simulink subsystem "Forces_and_Moments"  (R2025b)
settings: Solver=VariableStepAuto  StartTime=0.0  StopTime=10.0  RelTol=1e-3
undefined symbols (not defined in the file): canard_pos_r_mean, chute_drogue_drag, chute_drogue_time, chute_enable, chute_main_drag, chute_main_threshold, chute_main_time, rocket_diameter
settings Model: Creator=joedo  LastModifiedBy=jaiden

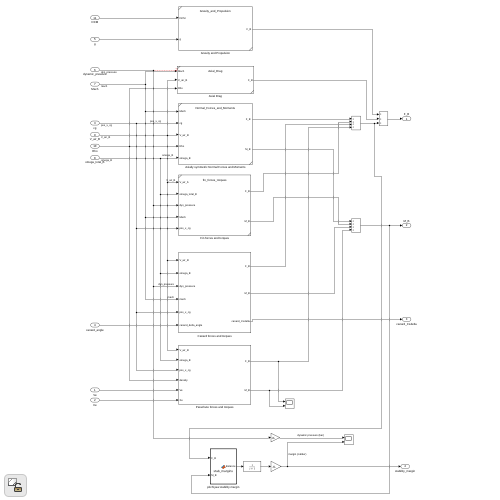
[thumbnail: Simulink's stored preview of the top-level diagram]
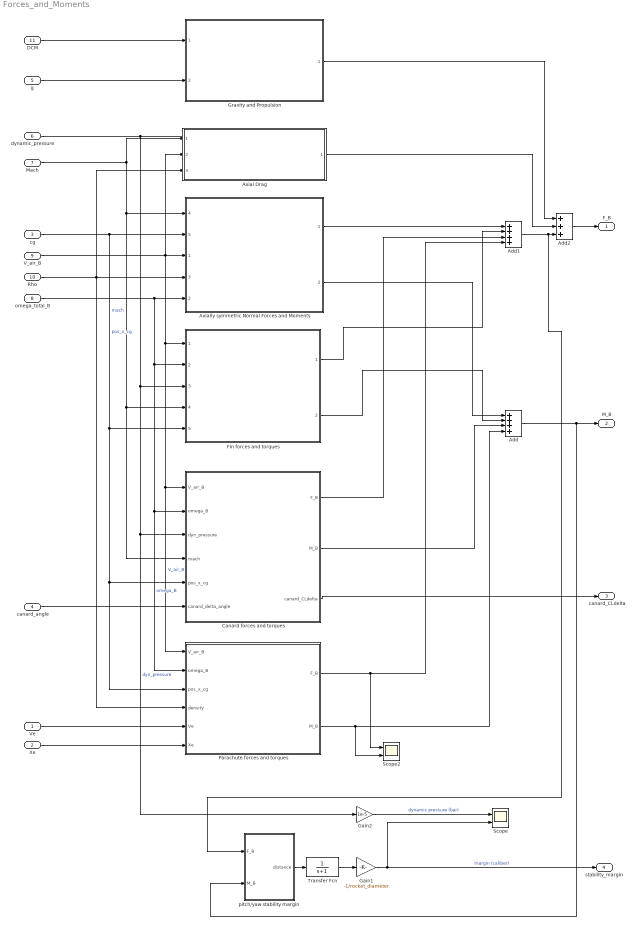
== system Forces_and_Moments ==
  Ve : Inport
  Xe : Inport  Port=2
  cg : Inport  Port=3
  canard_angle : Inport  Port=4
  g : Inport  Port=5
  "dynamic_pressure " : Inport  Port=6
  Mach : Inport  Port=7
  omega_total_B : Inport  Port=8
  V_air_B : Inport  Port=9
  Rho : Inport  Port=10
  DCM : Inport  Port=11
  Add : Sum  Inputs=++++
  Add1 : Sum  Inputs=++++
  Add2 : Sum  Inputs=+++
  Axial Drag : Subsystem  ReferencedSubsystem=Axial_Drag
  Axially symmetric Normal Forces and Moments : Subsystem  ReferencedSubsystem=Normal_Forces_and_Moments
      settings: PortSchema="{\"entries\":[{\"content\":{\"sides\":[{\"content\":{\"connectorIds\":[\"In4\",\"In5\",\"In1\",\"In3\",\"In2\"]},\"type\":\"ConnectorPlacement.EquallySpacedRectSide\",\"uuid\":\"3d060e6d-6cf3-4341-877b-3cb591774c08\"},{\"content\":{\"connectorIds\":[\"Out1\",\"Out2\"],\"side\":\"RIGHT\"},\"type\":\"ConnectorPlacement.EquallySpacedRectSide\",\"uuid\":\"12a83e93-0b1c-4946-a0d1-6eef9ce0d7d5\"},{\"content\":{\"side\":\"TOP\"},\"type\":\"ConnectorPlacement.EquallySpacedRectSide\",\"uuid\":\"237cf4f0-7c1b-4235-9d1e-c459b6944e6b\"}]},\"type\":\"ConnectorPlacement.EquallySpacedConnector\",\"uuid\":\"ee604e45-0548-4bf4-9ee4-77069ab5adfd\"}],\"packageUris\":[\"http://schema.mathworks.com/mf0/Connector/R2020b\"],\"version\":\"1.0\"}"
  Canard forces and torques : Subsystem
  Fin forces and torques : Subsystem  ReferencedSubsystem=fin_forces_torques
  Gain1 : Gain  Gain=-1/rocket_diameter
  Gain2 : Gain  Gain=1e-5
  Gravity and Propulsion : Subsystem  ReferencedSubsystem=Gravity_and_Propulsion
  Parachute forces and torques : Subsystem
  Scope : Scope  NumInputPorts=2
      settings: DataLoggingVariableName=ScopeData10
  Scope2 : Scope  NumInputPorts=2
      settings: ActiveDisplayYMinimum=-1249.89993  ActiveDisplayYMaximum=1249.98195  DataLoggingVariableName=ScopeData11
  Transfer Fcn : TransferFcn  Denominator=[1 1]
  pitch/yaw stability margin : MATLAB Function  TreatAsAtomicUnit=on
  F_B : Outport  VectorParamsAs1DForOutWhenUnconnected=off
  M_B : Outport  Port=2  VectorParamsAs1DForOutWhenUnconnected=off
  canard_CLdelta : Outport  Port=3
  stability_margin : Outport  Port=4
  wires:
  Rho/1 -> Axially symmetric Normal Forces and Moments/3, Parachute forces and torques/4("density "), Axial Drag/3
  Gravity and Propulsion/1 -> Add2/1
  DCM/1 -> Gravity and Propulsion/1
  Axial Drag/1 -> Add2/2
  Axially symmetric Normal Forces and Moments/1 -> Add1/1
  Axially symmetric Normal Forces and Moments/2 -> Add/1
  g/1 -> Gravity and Propulsion/2
  canard_angle/1 -> Canard forces and torques/6(canard_delta_angle)
  Canard forces and torques/2(M_B) -> Add/3
  Canard forces and torques/3(canard_CLdelta) -> canard_CLdelta/1
  Canard forces and torques/1(F_B) -> Add1/3
  pitch/yaw stability margin/1(distance) -> Transfer Fcn/1
  Add2/1 -> F_B/1
  Add1/1 -> Add2/3, pitch/yaw stability margin/1(F_B)
  Add/1 -> pitch/yaw stability margin/2(M_B), M_B/1
  Transfer Fcn/1 -> Gain1/1
  Gain1/1 -> Scope/2, stability_margin/1  "margin (caliber)"
  Gain2/1 -> Scope/1  "dynamic pressure (bar)"
  Parachute forces and torques/2(M_B) -> Scope2/2, Add/4
  Ve/1 -> Parachute forces and torques/5(Ve)
  Xe/1 -> Parachute forces and torques/6(Xe)
  Parachute forces and torques/1(F_B) -> Scope2/1, Add1/4
  V_air_B/1 -> Axially symmetric Normal Forces and Moments/1, Fin forces and torques/1, Parachute forces and torques/1(V_air_B), Canard forces and torques/1(V_air_B), Axial Drag/2  "V_air_B"
  Mach/1 -> Fin forces and torques/4, Canard forces and torques/4(mach), Axially symmetric Normal Forces and Moments/4, Axial Drag/1  "mach"
  cg/1 -> Fin forces and torques/5, Canard forces and torques/5(pos_x_cg), Parachute forces and torques/3(pos_x_cg), Axially symmetric Normal Forces and Moments/5  "pos_x_cg"
  "dynamic_pressure "/1 -> Fin forces and torques/3, Canard forces and torques/3(dyn_pressure), Gain2/1  "dyn_pressure"
  omega_total_B/1 -> Fin forces and torques/2, Canard forces and torques/2(omega_B), Parachute forces and torques/2(omega_B), Axially symmetric Normal Forces and Moments/2  "omega_B"
  Fin forces and torques/1 -> Add1/2
  Fin forces and torques/2 -> Add/2

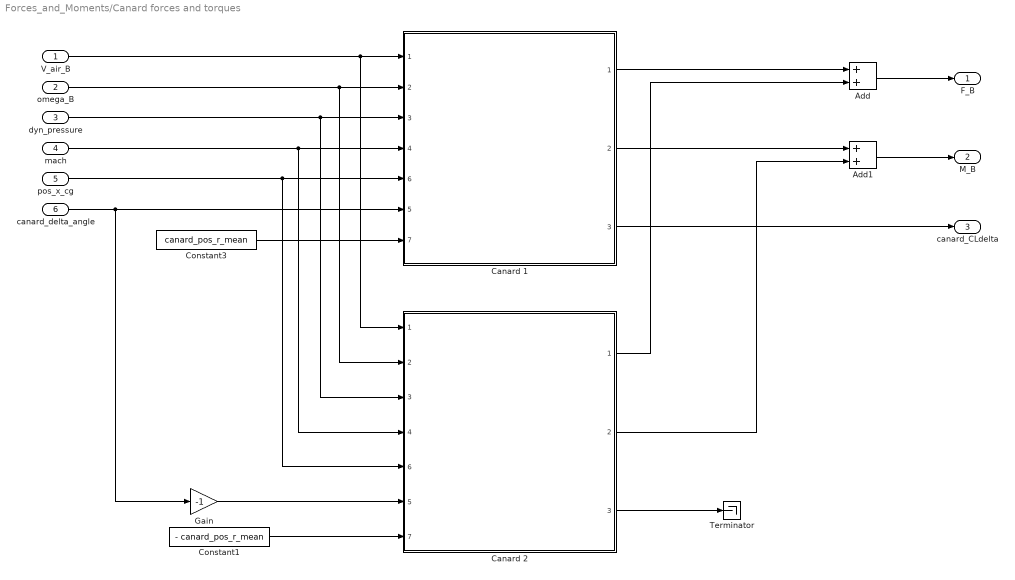
== system Forces_and_Moments/Canard forces and torques ==
  V_air_B : Inport
  omega_B : Inport  Port=2
  dyn_pressure : Inport  Port=3
  mach : Inport  Port=4
  pos_x_cg : Inport  Port=5
  canard_delta_angle : Inport  Port=6
  Add : Sum
  Add1 : Sum
  Canard 1 : Subsystem  ReferencedSubsystem=canard_forces_torques
      settings: PortSchema="{\"entries\":[{\"content\":{\"sides\":[{\"content\":{\"connectorIds\":[\"In1\",\"In2\",\"In3\",\"In4\",\"In6\",\"In5\",\"In7\"]},\"type\":\"ConnectorPlacement.EquallySpacedRectSide\",\"uuid\":\"f82ae2ae-cfd2-4bda-9eb8-bd0432545c6b\"},{\"content\":{\"connectorIds\":[\"Out1\",\"Out2\",\"Out3\"],\"side\":\"RIGHT\"},\"type\":\"ConnectorPlacement.EquallySpacedRectSide\",\"uuid\":\"6193b4bc-ea99-422c-bfe9-da5470a4c34b\"},{\"content\":{\"side\":\"TOP\"},\"type\":\"ConnectorPlacement.EquallySpacedRectSide\",\"uuid\":\"24e2ab5f-0d21-4ef4-a4c1-213001febe3d\"}]},\"type\":\"ConnectorPlacement.EquallySpacedConnector\",\"uuid\":\"07cc586d-e928-4dd6-ad4e-8adf17bfc056\"}],\"packageUris\":[\"http://schema.mathworks.com/mf0/Connector/R2020b\"],\"version\":\"1.0\"}"
  Canard 2 : Subsystem  ReferencedSubsystem=canard_forces_torques
      settings: PortSchema="{\"entries\":[{\"content\":{\"sides\":[{\"content\":{\"connectorIds\":[\"In1\",\"In2\",\"In3\",\"In4\",\"In6\",\"In5\",\"In7\"]},\"type\":\"ConnectorPlacement.EquallySpacedRectSide\",\"uuid\":\"f82ae2ae-cfd2-4bda-9eb8-bd0432545c6b\"},{\"content\":{\"connectorIds\":[\"Out1\",\"Out2\",\"Out3\"],\"side\":\"RIGHT\"},\"type\":\"ConnectorPlacement.EquallySpacedRectSide\",\"uuid\":\"6193b4bc-ea99-422c-bfe9-da5470a4c34b\"},{\"content\":{\"side\":\"TOP\"},\"type\":\"ConnectorPlacement.EquallySpacedRectSide\",\"uuid\":\"24e2ab5f-0d21-4ef4-a4c1-213001febe3d\"}]},\"type\":\"ConnectorPlacement.EquallySpacedConnector\",\"uuid\":\"07cc586d-e928-4dd6-ad4e-8adf17bfc056\"}],\"packageUris\":[\"http://schema.mathworks.com/mf0/Connector/R2020b\"],\"version\":\"1.0\"}"
  Constant1 : Constant  Value=- canard_pos_r_mean
  Constant3 : Constant  Value=canard_pos_r_mean
  Gain : Gain  Gain=-1
  Terminator : Terminator
  F_B : Outport
  M_B : Outport  Port=2
  canard_CLdelta : Outport  Port=3
  wires:
  Canard 1/3 -> canard_CLdelta/1
  pos_x_cg/1 -> Canard 2/6, Canard 1/6
  Add1/1 -> M_B/1
  Add/1 -> F_B/1
  Canard 2/3 -> Terminator/1
  Gain/1 -> Canard 2/5
  Canard 2/2 -> Add1/2
  Canard 1/1 -> Add/1
  canard_delta_angle/1 -> Canard 1/5, Gain/1
  omega_B/1 -> Canard 1/2, Canard 2/2
  V_air_B/1 -> Canard 1/1, Canard 2/1
  Canard 2/1 -> Add/2
  mach/1 -> Canard 1/4, Canard 2/4
  Canard 1/2 -> Add1/1
  Constant1/1 -> Canard 2/7
  Constant3/1 -> Canard 1/7
  dyn_pressure/1 -> Canard 1/3, Canard 2/3

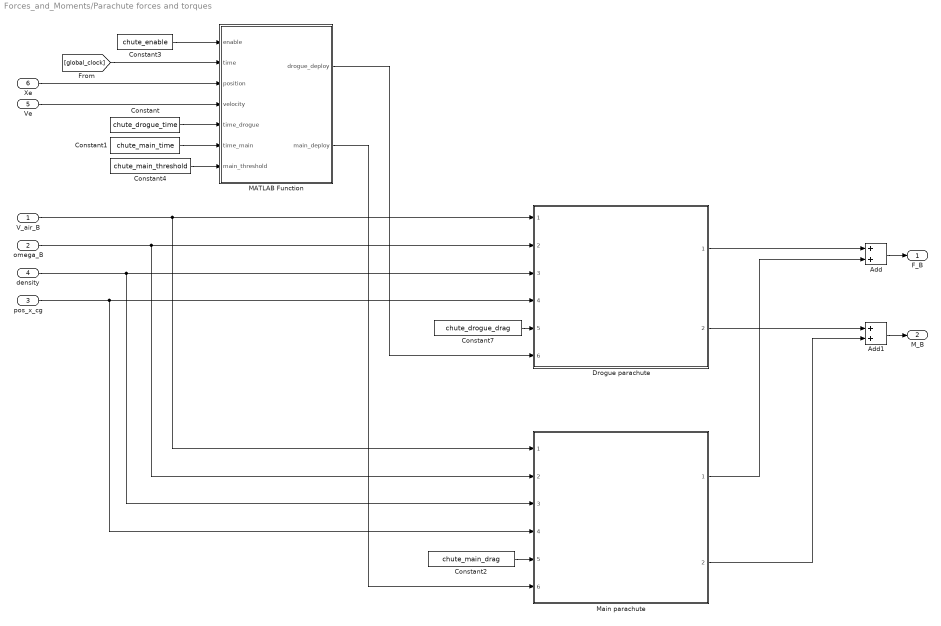
== system Forces_and_Moments/Parachute forces and torques ==
  V_air_B : Inport
  omega_B : Inport  Port=2
  pos_x_cg : Inport  Port=3
  "density " : Inport  Port=4
  Ve : Inport  Port=5
  Xe : Inport  Port=6
  Add : Sum
  Add1 : Sum
  Constant : Constant  Value=chute_drogue_time
  Constant1 : Constant  Value=chute_main_time
  Constant2 : Constant  Value=chute_main_drag
  Constant3 : Constant  Value=chute_enable
  Constant4 : Constant  Value=chute_main_threshold
  Constant7 : Constant  Value=chute_drogue_drag
  Drogue parachute : Subsystem  ReferencedSubsystem=chute_forces
  MATLAB Function : MATLAB Function  TreatAsAtomicUnit=on
  Main parachute : Subsystem  ReferencedSubsystem=chute_forces
  F_B : Outport
  M_B : Outport  Port=2
  wires:
  MATLAB Function/2(main_deploy) -> Main parachute/6
  MATLAB Function/1(drogue_deploy) -> Drogue parachute/6
  Constant4/1 -> MATLAB Function/7(main_threshold)
  Constant1/1 -> MATLAB Function/6(time_main)
  Constant/1 -> MATLAB Function/5(time_drogue)
  Xe/1 -> MATLAB Function/3(position)
  Ve/1 -> MATLAB Function/4(velocity)
  Constant3/1 -> MATLAB Function/1(enable)
  [global_clock] -> MATLAB Function/2(time)
  Add1/1 -> M_B/1
  Add/1 -> F_B/1
  Drogue parachute/2 -> Add1/1
  Main parachute/2 -> Add1/2
  Main parachute/1 -> Add/2
  Drogue parachute/1 -> Add/1
  Constant7/1 -> Drogue parachute/5
  pos_x_cg/1 -> Drogue parachute/4, Main parachute/4
  "density "/1 -> Drogue parachute/3, Main parachute/3
  V_air_B/1 -> Drogue parachute/1, Main parachute/1
  omega_B/1 -> Drogue parachute/2, Main parachute/2
  Constant2/1 -> Main parachute/5

== matlab function Forces_and_Moments/Parachute forces and torques/MATLAB Function ==
  data: drogue_deploy output; enable input; time input; main_deploy output; position input; velocity input; time_drogue input; time_main input; main_threshold input
function [drogue_deploy, main_deploy]  = deploy(enable, time, position, velocity, time_drogue, time_main, main_threshold)
    persistent t1 t2

    drogue_deploy = 0;
    main_deploy = 0;

    % drogue after apogee
    if enable(1) == 1 && velocity(1) < 0
        if isempty(t1)
            t1 = time;
        elseif time >= t1+time_drogue
            drogue_deploy = 1;
        end
    end

    % main after altitude
    if enable(2) == 1 && velocity(1) < 0 && position(1) <= main_threshold
        if isempty(t2)
            t2 = time;
        elseif time >= t2+time_main
            main_deploy = 1;
        end
    end
end

== matlab function Forces_and_Moments/pitch//yaw stability margin ==
  data: F_B input; M_B input; distance output
function distance  = stab_margins(F_B, M_B)
    
    % only absolute normal force, torque
    
    % project to x-normal plane
    F_yz = F_B(2:3);
    M_yz = M_B(2:3);

    % find magnitude and normal direction of net forces, moment
    F_mag = norm(F_yz);
    F_dir = atan2(F_yz(1), F_yz(2));
    M_mag = norm(M_yz);
    M_dir = atan2(M_yz(1), M_yz(2));
    
    % find main axes of force
    R = @(angle) [cos(angle), -sin(angle); sin(angle), cos(angle)];
    F_main = R(F_dir) * F_yz;
    M_main = R(F_dir) * M_yz;

    F = F_main(2);
    M = M_main(1);

    % exclude no force
    if F ~= 0
        distance = M / F;
    else 
        distance = -10; % arbitrary large value for no normal force
    end

end

% Body relative velocity magnitude
    % Vrel_mag = norm(Vrel);
    % Vrel_X = Vrel(1);
    % Vrel_magYZ = norm(Vrel(2:3));
    % 
    % incidence = atan2(Vrel_magYZ, Vrel_X);
